simulink model "simopt"  (Simulink 7.9)
settings: Solver=ode5  StartTime=0.0  StopTime=10  FixedStep=0.01  RelTol=1e-3
values from neighbouring files (symbols this model uses):
  Kd = K(3)    [FuncaoObjetivo.m]    (also in PIDcontrol.m = vecKs(3); opt_simopt.m = x(3); simopterror.m = x(3))
  Ki = K(2)    [FuncaoObjetivo.m]    (also in PIDcontrol.m = vecKs(2); opt_simopt.m = x(2); simopterror.m = x(2))
  Kp = K(1)    [FuncaoObjetivo.m]    (also in PIDcontrol.m = vecKs(1); opt_simopt.m = x(1); simopterror.m = x(1))
settings Model: Creator=Patcha  LastModifiedBy=Patcha  ExtModeTrigMode=oneshot  ExtModeArmWhenConnect=off
settings DataIOCC: LimitDataPoints=off  TimeSaveName=t  SignalLoggingName=sigsOut
settings OptimizationCC: BooleanDataType=off  InitFltsAndDblsToZero=on
settings DebuggingCC: SaveWithParameterizedLinksMsg=none  SignalResolutionControl=TryResolveAllWithWarning  SolverPrmCheckMsg=none  MultiTaskDSMMsg=warning  MultiTaskCondExecSysMsg=none  FcnCallInpInsideContextMsg=Use local settings  StrictBusMsg=None
settings HardwareCC: TargetUnknown=on
settings RTWCC: IncludeERTFirstTime=on
settings GRTTargetCC: TargetFcnLib=ansi_tfl_tmw.mat  CombineOutputUpdateFcns=off  GRTInterface=on

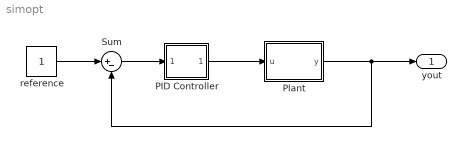
== system simopt ==
  PID Controller : Subsystem  mask(PID Controller){P=Kp, I=Ki, D=Kd}
      mask prompts: P "Proportional:"; I "Integral"; D "Derivative:"
      mask help:
      | Enter expressions for proportional, integral, and derivative terms.
      | P+I/s+Ds
      mask Help: This block implements a PID controller where parameters are entered for the Proportional, Integral and Derivative terms. Unmask this block to see how it works. The derivative term is implemented using a true derivative block.
      mask Display: disp('PID')
  Plant : Subsystem
  Sum : Sum  Inputs=|+-  SaturateOnIntegerOverflow=on  InputSameDT=on  OutDataTypeStr=Inherit: Same as first input
  reference : Constant
  yout : Outport
  wires:
  Sum/1 -> PID Controller/1(In_1)
  Plant/1(y) -> Sum/2, yout/1
  reference/1 -> Sum/1
  PID Controller/1(Out_1) -> Plant/1(u)

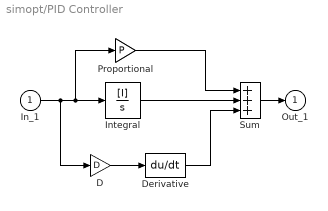
== system simopt/PID Controller ==
  In_1 : Inport
  D : Gain  Gain=D  SaturateOnIntegerOverflow=on  OutDataTypeStr=Inherit: Same as input  ParamDataTypeStr=Inherit: Same as input
  Derivative : Derivative
  Integral : TransferFcn  Numerator=[I]  Denominator=[1 0]
  Proportional : Gain  Gain=P  SaturateOnIntegerOverflow=on  OutDataTypeStr=Inherit: Same as input  ParamDataTypeStr=Inherit: Same as input
  Sum : Sum  Inputs=+++  SaturateOnIntegerOverflow=on  InputSameDT=on  OutDataTypeStr=Inherit: Same as first input
  Out_1 : Outport  InitialOutput=0
  wires:
  Proportional/1 -> Sum/1
  Integral/1 -> Sum/2
  Derivative/1 -> Sum/3
  In_1/1 -> Integral/1, Proportional/1, D/1
  Sum/1 -> Out_1/1
  D/1 -> Derivative/1

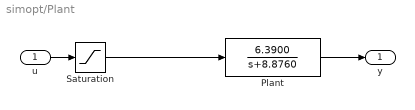
== system simopt/Plant ==
  u : Inport
  Plant : TransferFcn  Numerator=[6.3900]  Denominator=[1 8.8760]
  Saturation : Saturate  UpperLimit=12  LowerLimit=0
  y : Outport
  wires:
  Plant/1 -> y/1
  u/1 -> Saturation/1
  Saturation/1 -> Plant/1
